simulink model "proportional_NavSimulink"  (R2023b)
settings: Solver=ode1  StartTime=0.0  StopTime=inf  FixedStep=0.01  RelTol=1e-3
values from neighbouring files (symbols this model uses):
  Beta = 0.    (= 0)    [proportional_Nav.m]
  HE = HE * pi/180    (= -0.349065850399)    [proportional_Nav.m]
  R_Mx = coeff*(R_Mx_Old + H*V_Mx)    [proportional_Nav.m]
  R_My = coeff*(R_My_Old + H*V_My)    [proportional_Nav.m]
  R_Tx = coeff*(R_Tx_Old + H*V_Tx)    [proportional_Nav.m]
  R_Ty = coeff*(R_Ty_Old + H*V_Ty)    [proportional_Nav.m]
  V_M = 3000.    (= 3000)    [proportional_Nav.m]
  V_T = 1000.    (= 1000)    [proportional_Nav.m]
  XNP = 3.    (= 3)    [proportional_Nav.m]
  XNT = 96.6    [proportional_Nav.m]
libraries: simulink x2
settings Model: NumberOfSteps=15  Creator=hamdi  LastModifiedBy=hamdi
settings SolverCC: InitialStep=0.001  ZeroCrossAlgorithm=Adaptive

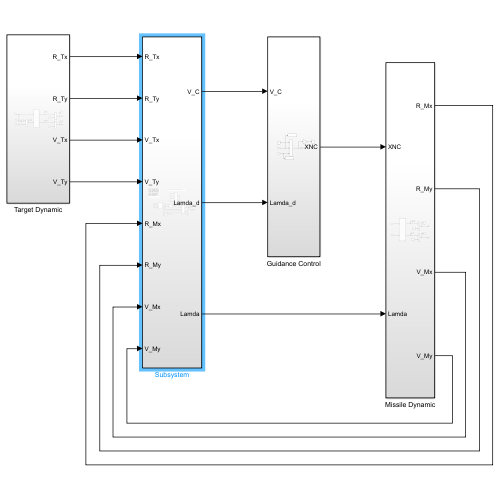
[thumbnail: Simulink's stored preview of the top-level diagram]
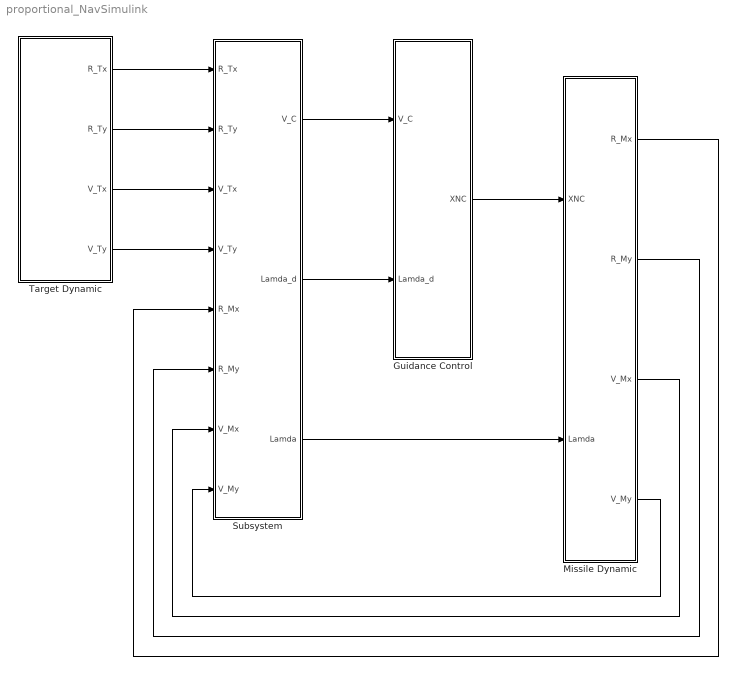
== system proportional_NavSimulink ==
  Guidance Control : Subsystem
  Missile Dynamic : Subsystem
  Subsystem : Subsystem
  Target Dynamic : Subsystem
  wires:
  Subsystem/1(V_C) -> Guidance Control/1(V_C)
  Subsystem/2(Lamda_d) -> Guidance Control/2(Lamda_d)
  Missile Dynamic/3(V_Mx) -> Subsystem/7(V_Mx)
  Missile Dynamic/4(V_My) -> Subsystem/8(V_My)
  Target Dynamic/3(V_Tx) -> Subsystem/3(V_Tx)
  Target Dynamic/4(V_Ty) -> Subsystem/4(V_Ty)
  Guidance Control/1(XNC) -> Missile Dynamic/1(XNC)
  Target Dynamic/1(R_Tx) -> Subsystem/1(R_Tx)
  Target Dynamic/2(R_Ty) -> Subsystem/2(R_Ty)
  Missile Dynamic/1(R_Mx) -> Subsystem/5(R_Mx)
  Missile Dynamic/2(R_My) -> Subsystem/6(R_My)
  Subsystem/3(Lamda) -> Missile Dynamic/2(Lamda)

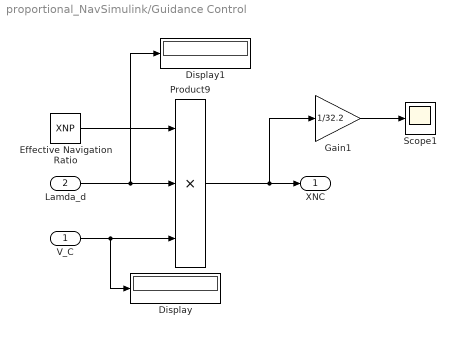
== system proportional_NavSimulink/Guidance Control ==
  V_C : Inport
  Lamda_d : Inport  Port=2
  Display : Display
  Display1 : Display
  "Effective Navigation Ratio " : Constant  Value=XNP
  Gain1 : Gain  Gain=1/32.2
  Product9 : Product  Inputs=3
  Scope1 : Scope
  XNC : Outport
  wires:
  V_C/1 -> Display/1, Product9/3
  "Effective Navigation Ratio "/1 -> Product9/1
  Lamda_d/1 -> Display1/1, Product9/2
  Product9/1 -> Gain1/1, XNC/1
  Gain1/1 -> Scope1/1

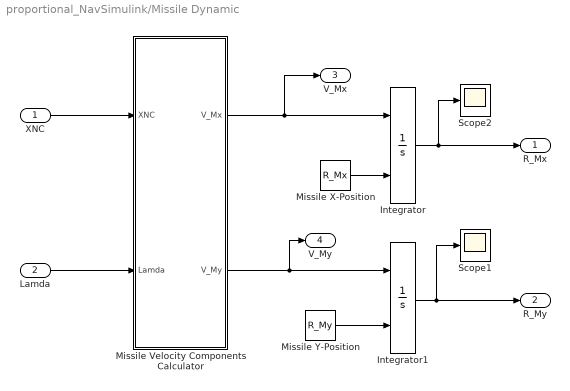
== system proportional_NavSimulink/Missile Dynamic ==
  XNC : Inport
  Lamda : Inport  Port=2
  Integrator : Integrator  InitialConditionSource=external
  Integrator1 : Integrator  InitialConditionSource=external
  Missile Velocity Components Calculator : Subsystem
  "Missile X-Position " : Constant  Value=R_Mx
  "Missile Y-Position " : Constant  Value=R_My
  Scope1 : Scope
  Scope2 : Scope
  R_Mx : Outport
  R_My : Outport  Port=2
  V_Mx : Outport  Port=3
  V_My : Outport  Port=4
  wires:
  "Missile X-Position "/1 -> Integrator/2
  "Missile Y-Position "/1 -> Integrator1/2
  Integrator/1 -> Scope2/1, R_Mx/1
  Integrator1/1 -> R_My/1, Scope1/1
  Missile Velocity Components Calculator/2(V_My) -> Integrator1/1, V_My/1
  Missile Velocity Components Calculator/1(V_Mx) -> V_Mx/1, Integrator/1
  XNC/1 -> Missile Velocity Components Calculator/1(XNC)
  Lamda/1 -> Missile Velocity Components Calculator/2(Lamda)

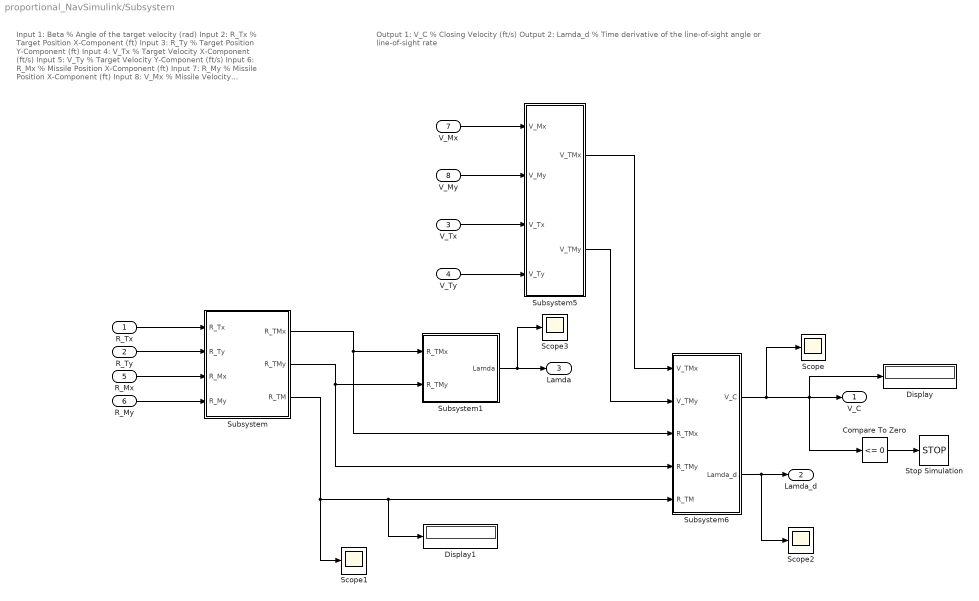
== system proportional_NavSimulink/Subsystem ==
  note: Output 1: V_C % Closing Velocity (ft/s)
      | Output 2: Lamda_d % Time derivative of the line-of-sight angle or line-of-sight rate
  note: Input 1: Beta % Angle of the target velocity (rad)
      | Input 2: R_Tx % Target Position X-Component (ft)
      | Input 3: R_Ty % Target Position Y-Component (ft)
      | Input 4: V_Tx % Target Velocity X-Component (ft/s)
      | Input 5: V_Ty % Target Velocity Y-Component (ft/s)
      | Input 6: R_Mx % Missile Position X-Component (ft)
      | Input 7: R_My % Missile Position X-Component (ft)
      | Input 8: V_Mx % Missile Velocity X-Component (ft/s)
      | Input 9: V_My % Missile Velocity X-Component (ft/s)
      | Input 10: V_M % Velocity of the missile (ft/s)
      | Input 11: V_T % Velocity of the target (ft/s)
      | Input 12: HE = HEDEG/57.3 % Heading error (rad)
      | Input 13: XNT % Target maneuver
      | Input 14: XNP % Effective navigation ratio or gain
  R_Tx : Inport
  R_Ty : Inport  Port=2
  V_Tx : Inport  Port=3
  V_Ty : Inport  Port=4
  R_Mx : Inport  Port=5
  R_My : Inport  Port=6
  V_Mx : Inport  Port=7
  V_My : Inport  Port=8
  Compare To Zero : simulink/Logic and Bit Operations/Compare To Zero  relop=<=  OutDataTypeStr=boolean
  Display : Display
  Display1 : Display
  Scope{,1..3} (4 alike) : Scope
  Stop Simulation : Stop
  Subsystem : Subsystem
  Subsystem1 : Subsystem
  Subsystem5 : Subsystem
  Subsystem6 : Subsystem
  V_C : Outport
  Lamda_d : Outport  Port=2
  Lamda : Outport  Port=3
  wires:
  Subsystem/1(R_TMx) -> Subsystem6/3(R_TMx), Subsystem1/1(R_TMx)
  Subsystem/2(R_TMy) -> Subsystem6/4(R_TMy), Subsystem1/2(R_TMy)
  Subsystem1/1(Lamda) -> Lamda/1, Scope3/1
  Subsystem5/1(V_TMx) -> Subsystem6/1(V_TMx)
  Subsystem5/2(V_TMy) -> Subsystem6/2(V_TMy)
  R_Tx/1 -> Subsystem/1(R_Tx)
  R_Mx/1 -> Subsystem/3(R_Mx)
  R_My/1 -> Subsystem/4(R_My)
  R_Ty/1 -> Subsystem/2(R_Ty)
  V_Ty/1 -> Subsystem5/4(V_Ty)
  V_Tx/1 -> Subsystem5/3(V_Tx)
  V_Mx/1 -> Subsystem5/1(V_Mx)
  V_My/1 -> Subsystem5/2(V_My)
  Compare To Zero/1 -> Stop Simulation/1
  Subsystem6/1(V_C) -> Scope/1, Compare To Zero/1, V_C/1, Display/1
  Subsystem/3(R_TM) -> Scope1/1, Display1/1, Subsystem6/5(R_TM)
  Subsystem6/2(Lamda_d) -> Scope2/1, Lamda_d/1

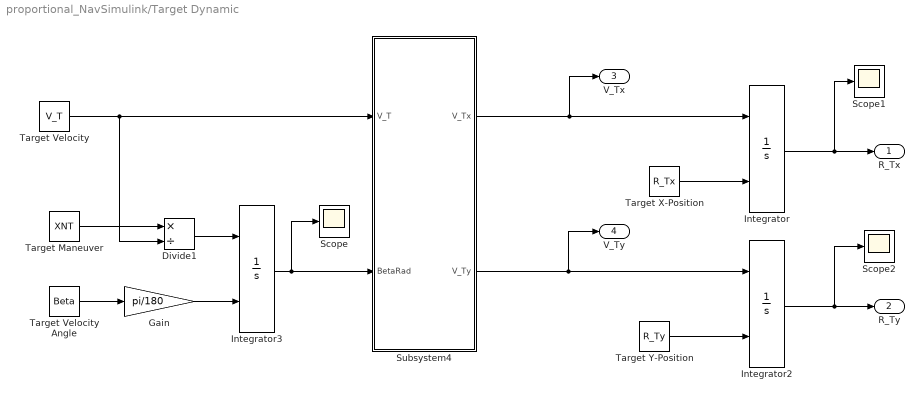
== system proportional_NavSimulink/Target Dynamic ==
  Divide1 : Product  Inputs=*/
  Gain : Gain  Gain=pi/180
  Integrator : Integrator  InitialConditionSource=external
  Integrator2 : Integrator  InitialConditionSource=external
  Integrator3 : Integrator  InitialConditionSource=external
  Scope : Scope
  Scope1 : Scope
  Scope2 : Scope
  Subsystem4 : Subsystem
  Target Maneuver : Constant  Value=XNT
  Target Velocity : Constant  Value=V_T
  Target Velocity Angle : Constant  Value=Beta
  "Target X-Position " : Constant  Value=R_Tx
  "Target Y-Position " : Constant  Value=R_Ty
  R_Tx : Outport
  R_Ty : Outport  Port=2
  V_Tx : Outport  Port=3
  V_Ty : Outport  Port=4
  wires:
  Target Velocity Angle/1 -> Gain/1
  Target Velocity/1 -> Divide1/2, Subsystem4/1(V_T)
  Divide1/1 -> Integrator3/1
  Subsystem4/2(V_Ty) -> V_Ty/1, Integrator2/1
  Subsystem4/1(V_Tx) -> V_Tx/1, Integrator/1
  Integrator3/1 -> Subsystem4/2(BetaRad), Scope/1
  Gain/1 -> Integrator3/2
  "Target X-Position "/1 -> Integrator/2
  "Target Y-Position "/1 -> Integrator2/2
  Integrator/1 -> Scope1/1, R_Tx/1
  Integrator2/1 -> Scope2/1, R_Ty/1
  Target Maneuver/1 -> Divide1/1

== system proportional_NavSimulink/Missile Dynamic/Missile Velocity Components Calculator ==
  XNC : Inport
  Lamda : Inport  Port=2
  Subsystem2 : Subsystem
  Subsystem3 : Subsystem
  V_Mx : Outport
  V_My : Outport  Port=2
  wires:
  Subsystem3/2(V_My) -> V_My/1
  Lamda/1 -> Subsystem3/1(Lamda)
  Subsystem2/2(V_My0) -> Subsystem3/4(V_My0)
  Subsystem2/1(V_Mx0) -> Subsystem3/3(V_Mx0)
  XNC/1 -> Subsystem3/2(XNC)
  Subsystem3/1(V_Mx) -> V_Mx/1

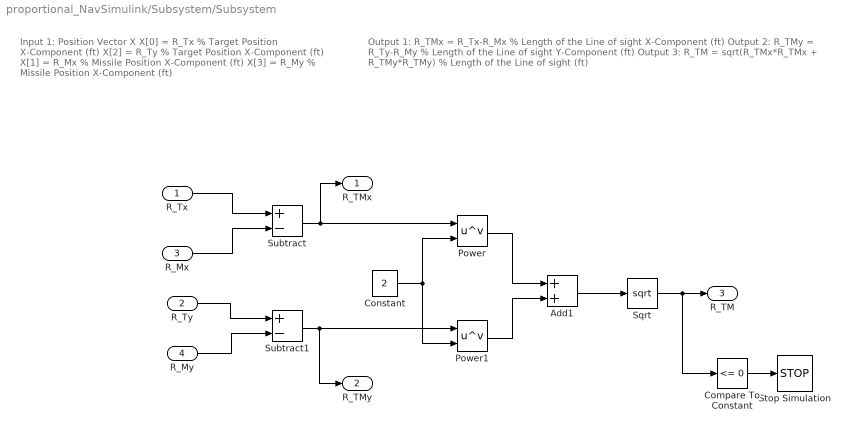
== system proportional_NavSimulink/Subsystem/Subsystem ==
  note: Output 1: R_TMx = R_Tx-R_Mx % Length of the Line of sight X-Component (ft)
      | Output 2: R_TMy = R_Ty-R_My % Length of the Line of sight Y-Component (ft)
      | Output 3: R_TM = sqrt(R_TMx*R_TMx + R_TMy*R_TMy) % Length of the Line of sight (ft)
  note: Input 1: Position Vector X
      | X[0] = R_Tx % Target Position X-Component (ft)
      | X[2] = R_Ty % Target Position X-Component (ft)
      | X[1] = R_Mx % Missile Position X-Component (ft)
      | X[3] = R_My % Missile Position X-Component (ft)
  R_Tx : Inport
  R_Ty : Inport  Port=2
  R_Mx : Inport  Port=3
  R_My : Inport  Port=4
  Add1 : Sum
  Compare To Constant : simulink/Logic and Bit Operations/Compare To Constant  relop=<=  const=0  OutDataTypeStr=boolean
  Constant : Constant  Value=2
  Power : Math  Operator=pow
  Power1 : Math  Operator=pow
  Sqrt : Sqrt
  Stop Simulation : Stop
  Subtract : Sum  Inputs=+-
  Subtract1 : Sum  Inputs=+-
  R_TMx : Outport
  R_TMy : Outport  Port=2
  R_TM : Outport  Port=3
  wires:
  Subtract1/1 -> Power1/1, R_TMy/1
  Constant/1 -> Power1/2, Power/2
  Power1/1 -> Add1/2
  Add1/1 -> Sqrt/1
  Power/1 -> Add1/1
  Subtract/1 -> Power/1, R_TMx/1
  R_Ty/1 -> Subtract1/1
  R_My/1 -> Subtract1/2
  R_Mx/1 -> Subtract/2
  R_Tx/1 -> Subtract/1
  Sqrt/1 -> Compare To Constant/1, R_TM/1
  Compare To Constant/1 -> Stop Simulation/1

== system proportional_NavSimulink/Subsystem/Subsystem1 ==
  note: Input 1: R_TMx % Length of the Line of sight X-Component (ft)
      | Input 2: R_TMy % Length of the Line of sight Y-Component (ft)
  note: Output 1: Lamda = atan2(R_TMy,R_TMx) % Line-of-sight angle (rad)
  R_TMx : Inport
  R_TMy : Inport  Port=2
  Atan2 : Trigonometry  Operator=atan2
  Lamda : Outport
  wires:
  Atan2/1 -> Lamda/1
  R_TMx/1 -> Atan2/2
  R_TMy/1 -> Atan2/1

== system proportional_NavSimulink/Subsystem/Subsystem5 ==
  note: Input 1: V_Mx % Missile velocity X-Component (ft/s)
      | Input 2: V_My % Missile velocity Y-Component (ft/s)
      | Input 3: V_Tx % Target velocity X-Component (ft/s)
      | Input 4: V_Ty % Target velocity Y-Component (ft/s)
  note: Output 1: V_TMx = V_Tx - V_Mx % Velocity of the Line of sight X-Component (ft/s)
      | Output 2: V_TMy = V_Ty - V_My % Velocity of the Line of sight Y-Component (ft/s)
  V_Mx : Inport
  V_My : Inport  Port=2
  V_Tx : Inport  Port=3
  V_Ty : Inport  Port=4
  Subtract2 : Sum  Inputs=+-
  Subtract3 : Sum  Inputs=+-
  V_TMx : Outport
  V_TMy : Outport  Port=2
  wires:
  V_Ty/1 -> Subtract3/1
  V_Mx/1 -> Subtract2/2
  V_My/1 -> Subtract3/2
  V_Tx/1 -> Subtract2/1
  Subtract2/1 -> V_TMx/1
  Subtract3/1 -> V_TMy/1

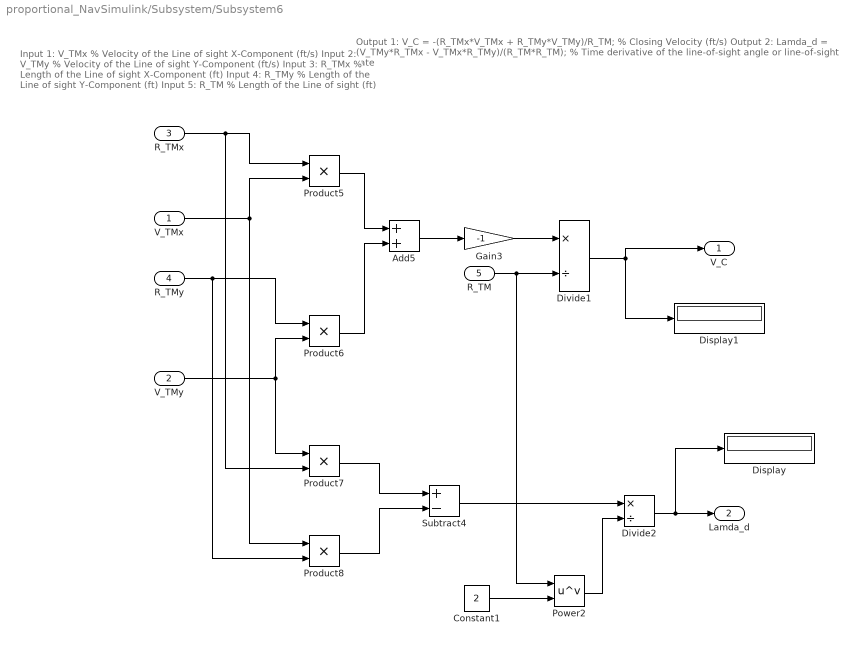
== system proportional_NavSimulink/Subsystem/Subsystem6 ==
  note: Output 1: V_C = -(R_TMx*V_TMx + R_TMy*V_TMy)/R_TM; % Closing Velocity (ft/s)
      | Output 2: Lamda_d = (V_TMy*R_TMx - V_TMx*R_TMy)/(R_TM*R_TM); % Time derivative of the line-of-sight angle or line-of-sight rate
  note: Input 1: V_TMx % Velocity of the Line of sight X-Component (ft/s)
      | Input 2: V_TMy % Velocity of the Line of sight Y-Component (ft/s)
      | Input 3: R_TMx % Length of the Line of sight X-Component (ft)
      | Input 4: R_TMy % Length of the Line of sight Y-Component (ft)
      | Input 5: R_TM % Length of the Line of sight (ft)
  V_TMx : Inport
  V_TMy : Inport  Port=2
  R_TMx : Inport  Port=3
  R_TMy : Inport  Port=4
  R_TM : Inport  Port=5
  Add5 : Sum
  Constant1 : Constant  Value=2
  Display : Display
  Display1 : Display
  Divide1 : Product  Inputs=*/
  Divide2 : Product  Inputs=*/
  Gain3 : Gain  Gain=-1
  Power2 : Math  Operator=pow
  Product{5..8} (4 alike) : Product
  Subtract4 : Sum  Inputs=+-
  V_C : Outport
  Lamda_d : Outport  Port=2
  wires:
  R_TMy/1 -> Product6/1, Product8/2
  Add5/1 -> Gain3/1
  R_TM/1 -> Power2/1, Divide1/2
  R_TMx/1 -> Product5/1, Product7/2
  V_TMx/1 -> Product8/1, Product5/2
  Product6/1 -> Add5/2
  V_TMy/1 -> Product7/1, Product6/2
  Product5/1 -> Add5/1
  Subtract4/1 -> Divide2/1
  Power2/1 -> Divide2/2
  Product8/1 -> Subtract4/2
  Divide2/1 -> Display/1, Lamda_d/1
  Product7/1 -> Subtract4/1
  Constant1/1 -> Power2/2
  Divide1/1 -> Display1/1, V_C/1
  Gain3/1 -> Divide1/1

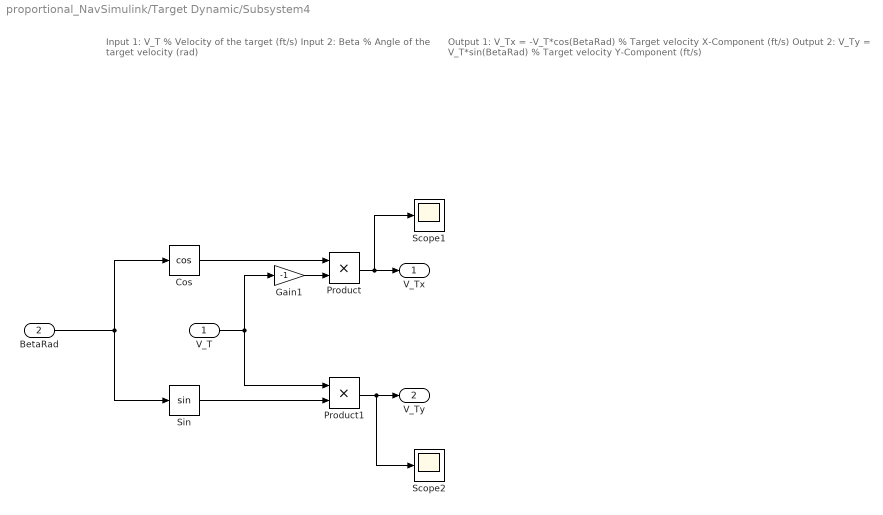
== system proportional_NavSimulink/Target Dynamic/Subsystem4 ==
  note: Input 1: V_T % Velocity of the target (ft/s)
      | Input 2: Beta % Angle of the target velocity (rad)
  note: Output 1: V_Tx = -V_T*cos(BetaRad) % Target velocity X-Component (ft/s)
      | Output 2: V_Ty = V_T*sin(BetaRad) % Target velocity Y-Component (ft/s)
  V_T : Inport
  BetaRad : Inport  Port=2
  Cos : Trigonometry  Operator=cos
  Gain1 : Gain  Gain=-1
  Product : Product
  Product1 : Product
  Scope1 : Scope
  Scope2 : Scope
  Sin : Trigonometry
  V_Tx : Outport
  V_Ty : Outport  Port=2
  wires:
  V_T/1 -> Product1/1, Gain1/1
  Gain1/1 -> Product/2
  Cos/1 -> Product/1
  BetaRad/1 -> Sin/1, Cos/1
  Sin/1 -> Product1/2
  Product/1 -> Scope1/1, V_Tx/1
  Product1/1 -> Scope2/1, V_Ty/1

== system proportional_NavSimulink/Missile Dynamic/Missile Velocity Components Calculator/Subsystem2 ==
  Gain2 : Gain  Gain=pi/180
  Heading Error1 : Constant  Value=HE
  Missile Velocity : Constant  Value=V_M
  Subsystem : Subsystem
  Subsystem1 : Subsystem
  V_Mx0 : Outport
  V_My0 : Outport  Port=2
  wires:
  Subsystem1/1(Theta) -> Subsystem/1(Theta)
  Missile Velocity/1 -> Subsystem/2(V_M)
  Heading Error1/1 -> Gain2/1
  Gain2/1 -> Subsystem/3(HE)
  Subsystem/2(V_My0) -> V_My0/1
  Subsystem/1(V_Mx0) -> V_Mx0/1

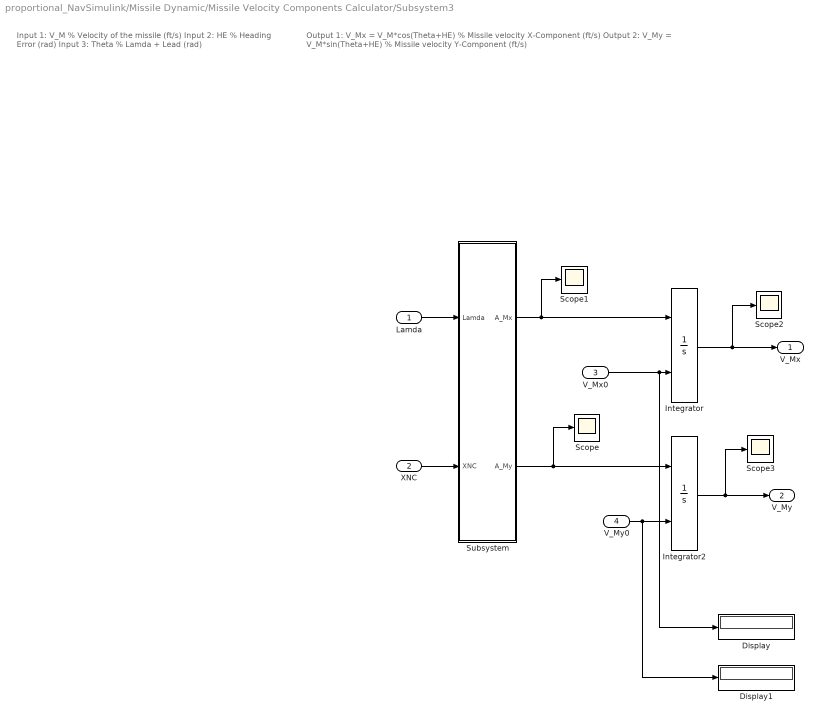
== system proportional_NavSimulink/Missile Dynamic/Missile Velocity Components Calculator/Subsystem3 ==
  note: Input 1: V_M % Velocity of the missile (ft/s)
      | Input 2: HE % Heading Error (rad)
      | Input 3: Theta % Lamda + Lead (rad)
  note: Output 1: V_Mx = V_M*cos(Theta+HE) % Missile velocity X-Component (ft/s)
      | Output 2: V_My = V_M*sin(Theta+HE) % Missile velocity Y-Component (ft/s)
  Lamda : Inport
  XNC : Inport  Port=2
  V_Mx0 : Inport  Port=3
  V_My0 : Inport  Port=4
  Display : Display
  Display1 : Display
  Integrator : Integrator  InitialConditionSource=external
  Integrator2 : Integrator  InitialConditionSource=external
  Scope{,1..3} (4 alike) : Scope
  Subsystem : Subsystem
  V_Mx : Outport
  V_My : Outport  Port=2
  wires:
  Integrator/1 -> Scope2/1, V_Mx/1
  Integrator2/1 -> V_My/1, Scope3/1
  V_My0/1 -> Integrator2/2, Display1/1
  V_Mx0/1 -> Display/1, Integrator/2
  Subsystem/1(A_Mx) -> Integrator/1, Scope1/1
  Subsystem/2(A_My) -> Integrator2/1, Scope/1
  Lamda/1 -> Subsystem/1(Lamda)
  XNC/1 -> Subsystem/2(XNC)

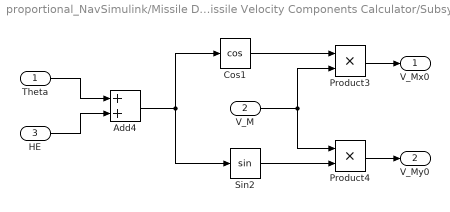
== system proportional_NavSimulink/Missile Dynamic/Missile Velocity Components Calculator/Subsystem2/Subsystem ==
  Theta : Inport
  V_M : Inport  Port=2
  HE : Inport  Port=3
  Add4 : Sum
  Cos1 : Trigonometry  Operator=cos
  Product3 : Product
  Product4 : Product
  Sin2 : Trigonometry
  V_Mx0 : Outport
  V_My0 : Outport  Port=2
  wires:
  Product4/1 -> V_My0/1
  Product3/1 -> V_Mx0/1
  Cos1/1 -> Product3/1
  Add4/1 -> Sin2/1, Cos1/1
  V_M/1 -> Product4/1, Product3/2
  Sin2/1 -> Product4/2
  Theta/1 -> Add4/1
  HE/1 -> Add4/2

== system proportional_NavSimulink/Missile Dynamic/Missile Velocity Components Calculator/Subsystem2/Subsystem1 ==
  Add1 : Sum
  Subsystem : Subsystem
  Subsystem1 : Subsystem
  Theta : Outport
  wires:
  Add1/1 -> Theta/1
  Subsystem/1(Lamda) -> Subsystem1/1(Lamda), Add1/1
  Subsystem1/1(Lead) -> Add1/2

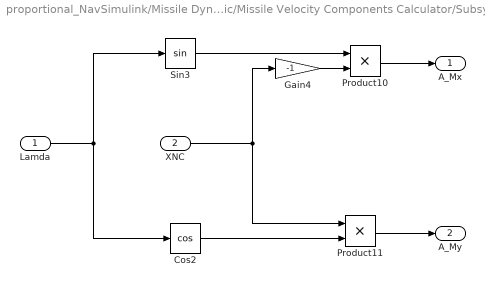
== system proportional_NavSimulink/Missile Dynamic/Missile Velocity Components Calculator/Subsystem3/Subsystem ==
  Lamda : Inport
  XNC : Inport  Port=2
  Cos2 : Trigonometry  Operator=cos
  Gain4 : Gain  Gain=-1
  Product10 : Product
  Product11 : Product
  Sin3 : Trigonometry
  A_Mx : Outport
  A_My : Outport  Port=2
  wires:
  XNC/1 -> Gain4/1, Product11/1
  Sin3/1 -> Product10/1
  Lamda/1 -> Cos2/1, Sin3/1
  Cos2/1 -> Product11/2
  Product11/1 -> A_My/1
  Gain4/1 -> Product10/2
  Product10/1 -> A_Mx/1

== system proportional_NavSimulink/Missile Dynamic/Missile Velocity Components Calculator/Subsystem2/Subsystem1/Subsystem ==
  Atan2 : Trigonometry  Operator=atan2
  Constant1 : Constant  Value=R_Tx
  Constant2 : Constant  Value=R_Ty
  Constant3 : Constant  Value=R_Mx
  Constant4 : Constant  Value=R_My
  Subtract : Sum  Inputs=+-
  Subtract1 : Sum  Inputs=+-
  Lamda : Outport
  wires:
  Constant3/1 -> Subtract/2
  Subtract1/1 -> Atan2/1
  Constant1/1 -> Subtract/1
  Constant4/1 -> Subtract1/2
  Subtract/1 -> Atan2/2
  Constant2/1 -> Subtract1/1
  Atan2/1 -> Lamda/1

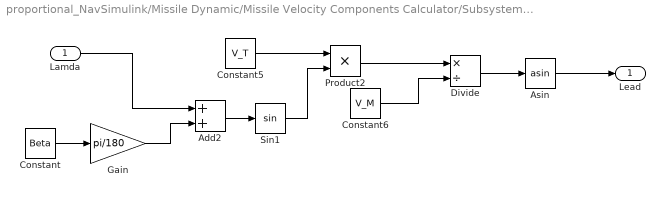
== system proportional_NavSimulink/Missile Dynamic/Missile Velocity Components Calculator/Subsystem2/Subsystem1/Subsystem1 ==
  Lamda : Inport
  Add2 : Sum
  Asin : Trigonometry  Operator=asin
  Constant : Constant  Value=Beta
  Constant5 : Constant  Value=V_T
  Constant6 : Constant  Value=V_M
  Divide : Product  Inputs=*/
  Gain : Gain  Gain=pi/180
  Product2 : Product
  Sin1 : Trigonometry
  Lead : Outport
  wires:
  Gain/1 -> Add2/2
  Add2/1 -> Sin1/1
  Constant6/1 -> Divide/2
  Constant5/1 -> Product2/1
  Sin1/1 -> Product2/2
  Divide/1 -> Asin/1
  Product2/1 -> Divide/1
  Constant/1 -> Gain/1
  Asin/1 -> Lead/1
  Lamda/1 -> Add2/1
